simulink model "motor1"  (R2020b)
settings: Solver=ode45  StartTime=0.0  StopTime=5  RelTol=1e-3  EnableMultiTasking=on
PreLoadFcn:
  | MotorParam
InitFcn:
  | MotorParam
values from neighbouring files (symbols this model uses):
  B = (Km*INL)/w    (= 4.14319136746e-07)    [MotorParam.m]
  J = Rotor_inertia    (= 2.23668e-07)    [MotorParam.m]
  Kb = (Speed_constant)/(.10472)    (= 0.0177826336223)    [MotorParam.m]
  Km = Torque_constant*1E-3    (= 0.0178)    [MotorParam.m]
  L = Terminal_inductance*1E-3    (= 0.000411)    [MotorParam.m]
  R = Terminal_resistance    (= 5.82)    [MotorParam.m]
settings Model: Creator=Leo  LastModifiedBy=Jeff
settings DataIOCC: LimitDataPoints=on  SaveFormat=Array  SignalLoggingSaveFormat=ModelDataLogs  ReturnWorkspaceOutputs=off
settings OptimizationCC: ExpressionDepthLimit=2147483647  InitFltsAndDblsToZero=on  LifeSpan=inf
settings DebuggingCC: UnderspecifiedInitializationDetection=Classic  MergeDetectMultiDrivingBlocksExec=none  SolverPrmCheckMsg=warning  FcnCallInpInsideContextMsg=warning  StateNameClashWarn=warning  SFUnexpectedBacktrackingDiag=warning  SFNoUnconditionalDefaultTransitionDiag=warning  SFExecutionAtInitializationDiag=none  ArithmeticOperatorsInVariantConditions=warning
settings HardwareCC: ProdBitPerPointer=32  ProdBitPerSizeT=32  ProdBitPerPtrDiffT=32  ProdLargestAtomicFloat=None  ProdIntDivRoundTo=Undefined  ProdEndianess=Unspecified  ProdWordSize=32  ProdHWDeviceType=32-bit Generic
settings ModelReferenceCC: PropagateSignalLabelsOutOfModel=off
settings SFSimCC: SimUseLocalCustomCode=off  CustomCodeUndefinedFunction=UseInterfaceOnly
settings RTWCC: RTWUseLocalCustomCode=off
settings CodeAppCC: StateflowObjectComments=on
settings GRTTargetCC: TargetLangStandard=C89/C90 (ANSI)  CombineOutputUpdateFcns=off  GRTInterface=on
settings ConfigComp: CovMetricSettings=dw  CovSaveCumulativeToWorkspaceVar=on  CovSaveSingleToWorkspaceVar=on  CovExternalEMLEnable=off  CovSFcnEnable=off

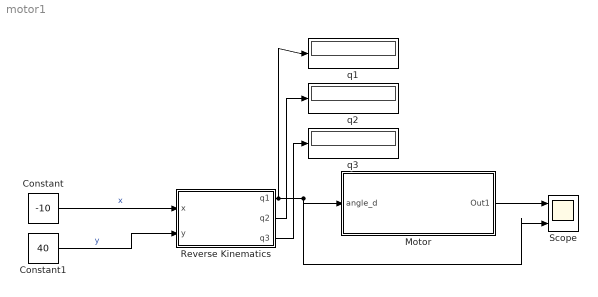
== system motor1 ==
  Constant : Constant  Value=-10
  Constant1 : Constant  Value=40
  Motor : Subsystem
  Reverse Kinematics : MATLAB Function  TreatAsAtomicUnit=on
  Scope : Scope  NumInputPorts=2
  q1 : Display
  q2 : Display
  q3 : Display
  wires:
  Constant/1 -> Reverse Kinematics/1(x)  "x"
  Motor/1(Out1) -> Scope/1
  Constant1/1 -> Reverse Kinematics/2(y)  "y"
  Reverse Kinematics/1(q1) -> q1/1, Motor/1(angle_d), Scope/2
  Reverse Kinematics/2(q2) -> q2/1
  Reverse Kinematics/3(q3) -> q3/1

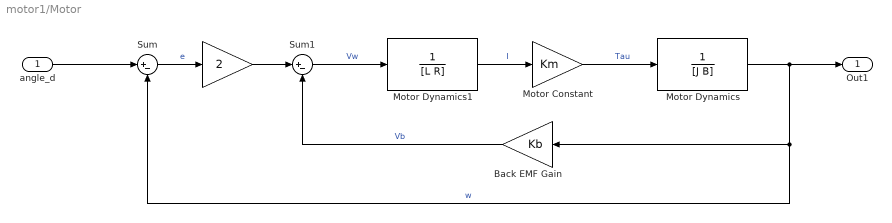
== system motor1/Motor ==
  angle_d : Inport
  " " : Gain  Gain=2
  Back EMF Gain : Gain  Gain=Kb
  Motor Constant : Gain  Gain=Km
  Motor Dynamics : TransferFcn  Denominator=[J B]
  Motor Dynamics1 : TransferFcn  Denominator=[L R]
  Sum : Sum  Inputs=|+-
  Sum1 : Sum  Inputs=|+-
  Out1 : Outport
  wires:
  angle_d/1 -> Sum/1
  Sum/1 -> " "/1  "e"
  Motor Dynamics/1 -> Out1/1, Sum/2, Back EMF Gain/1  "w"
  Motor Constant/1 -> Motor Dynamics/1  "Tau"
  " "/1 -> Sum1/1
  Back EMF Gain/1 -> Sum1/2  "Vb"
  Motor Dynamics1/1 -> Motor Constant/1  "I"
  Sum1/1 -> Motor Dynamics1/1  "Vw"

== matlab function motor1/Reverse Kinematics ==
  data: x input; q1 output; y input; q2 output; q3 output
% function [q1, q2, q3]= fcn(x,y)
%     l1 = 20;
%     l2 = 30;
%     
%     q2 = acosd((x^2+y^2-l1^2-l2^2)/(2*l1*l2));
%     q1 = atand(y/x)-asind(l2*sind(q2)/sqrt(x^2+y^2));
%     if q1<0 
%         q1 = 180+q1;
%     end
%     q3 = 180-q1-q2;
    
    function [q1, q2, q3]= fcn(x,y)
    a1 = 20;
    a2 = 30;
    
    q2 = acosd((x^2+y^2-a1^2-a2^2)/(2*a1*a2));
    q1 = atand(y/x)-atand(a2*sind(q2)/(a1+a2*cosd(q2)));
    if q1<0 
        q1 = 180+q1;
    end
    q3 = 180-q1-q2;
